simulink model "C2_sensor_backemf"  (Simulink 10.2)
settings: Solver=ode4  StartTime=0.0  StopTime=3  FixedStep=T_s  RelTol=1e-3
undefined symbols (not defined in the file): b_eq, beta_p, beta_v, g, i_rated, J_eq, k, L, L_l, m_l, N_adc, N_e, N_opt, R, R_sh, T_s, tau_m_rated, theta_0, V_adc
libraries: simulink x1
settings Model: Creator=ioannis  LastModifiedBy=mfocchi
settings DataIOCC: SaveFormat=Dataset  SignalLoggingSaveFormat=Dataset
settings OptimizationCC: LifeSpan=auto
settings DebuggingCC: UnderspecifiedInitializationDetection=Simplified  MergeDetectMultiDrivingBlocksExec=error  FcnCallInpInsideContextMsg=error  SFUnexpectedBacktrackingDiag=error  SFNoUnconditionalDefaultTransitionDiag=error  SFExecutionAtInitializationDiag=warning
settings HardwareCC: ProdBitPerPointer=64  ProdBitPerSizeT=64  ProdBitPerPtrDiffT=64  ProdLargestAtomicFloat=Float  ProdIntDivRoundTo=Zero  ProdEndianess=LittleEndian  ProdWordSize=64  ProdHWDeviceType=Intel->x86-64 (Windows64)
settings ModelReferenceCC: PropagateSignalLabelsOutOfModel=on
settings SFSimCC: SimUseLocalCustomCode=on
settings RTWCC: RTWUseLocalCustomCode=on
settings CodeAppCC: StateflowObjectComments=off
settings GRTTargetCC: TargetLangStandard=C99 (ISO)  CombineOutputUpdateFcns=on  GRTInterface=off
settings ConfigComp: CovMetricSettings=dwe  CovSaveCumulativeToWorkspaceVar=off  CovSaveSingleToWorkspaceVar=off  CovExternalEMLEnable=on

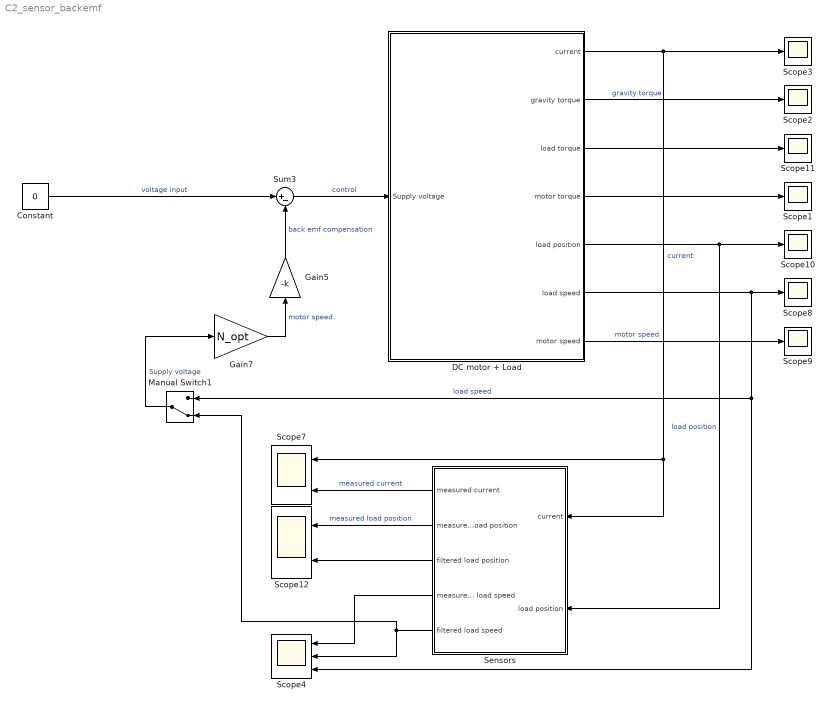
== system C2_sensor_backemf ==
  Constant : Constant  Value=0
  DC motor + Load : Subsystem
  Gain5 : Gain  Gain=-k
  Gain7 : Gain  Gain=N_opt
  Manual Switch1 : ManualSwitch  CurrentSetting=0
  Scope{1..3,8..11} (7 alike) : Scope
  Scope12 : Scope  NumInputPorts=2
  Scope4 : Scope  NumInputPorts=3
  Scope7 : Scope  NumInputPorts=2
  Sensors : Subsystem
  Sum3 : Sum  Inputs=|+-
  wires:
  DC motor + Load/6(load speed) -> Scope8/1, Scope4/3, Manual Switch1/1  "load speed"
  Sum3/1 -> DC motor + Load/1(Supply voltage)  "control"
  DC motor + Load/2(gravity torque) -> Scope2/1  "gravity torque"
  DC motor + Load/5(load position) -> Sensors/2(load position), Scope10/1  "load position"
  DC motor + Load/7(motor speed) -> Scope9/1  "motor speed"
  DC motor + Load/1(current) -> Sensors/1(current), Scope7/1, Scope3/1  "current"
  Constant/1 -> Sum3/1  "voltage input"
  DC motor + Load/3(load torque) -> Scope11/1
  DC motor + Load/4(motor torque) -> Scope1/1
  Sensors/2(measured load position) -> Scope12/1  "measured load position"
  Sensors/3(filtered load position) -> Scope12/2
  Sensors/4(measured load speed) -> Scope4/1
  Gain7/1 -> Gain5/1  "motor speed"
  Manual Switch1/1 -> Gain7/1  "Supply voltage"
  Sensors/5(filtered load speed) -> Scope4/2, Manual Switch1/2
  Sensors/1(measured current) -> Scope7/2  "measured current"
  Gain5/1 -> Sum3/2  "back emf compensation"

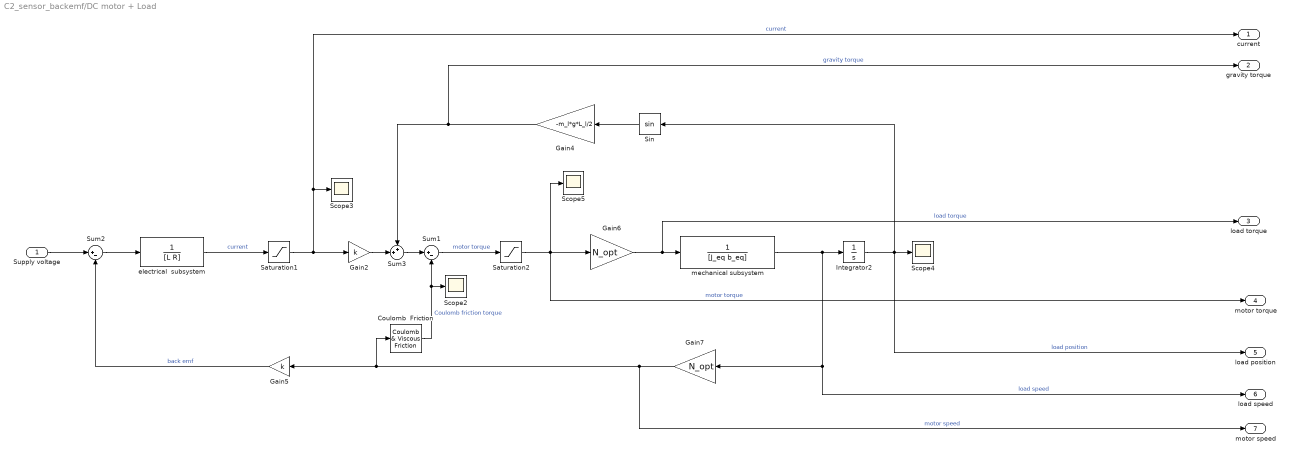
== system C2_sensor_backemf/DC motor + Load ==
  Supply voltage : Inport
  Coulomb  Friction : simulink/Discontinuities/Coulomb & Viscous Friction  offset=tau_c  gain=0
  Gain2 : Gain  Gain=k
  Gain4 : Gain  Gain=-m_l*g*L_l/2
  Gain5 : Gain  Gain=k
  Gain6 : Gain  Gain=N_opt
  Gain7 : Gain  Gain=N_opt
  Integrator2 : Integrator  InitialCondition=theta_0
  Saturation1 : Saturate  UpperLimit=i_rated  LowerLimit=-i_rated
  Saturation2 : Saturate  UpperLimit=tau_m_rated  LowerLimit=-tau_m_rated
  Scope{2..5} (4 alike) : Scope
  Sin : Trigonometry
  Sum1 : Sum  Inputs=|+-
  Sum2 : Sum  Inputs=|+-
  Sum3 : Sum  Inputs=++|
  electrical  subsystem : TransferFcn  Denominator=[L R]
  mechanical subsystem : TransferFcn  Denominator=[J_eq b_eq]
  current : Outport
  gravity torque : Outport  Port=2
  load torque : Outport  Port=3
  motor torque : Outport  Port=4
  load position : Outport  Port=5
  load speed : Outport  Port=6
  motor speed : Outport  Port=7
  wires:
  Sum2/1 -> electrical  subsystem/1
  Saturation2/1 -> motor torque/1, Scope5/1, Gain6/1  "motor torque"
  Sum3/1 -> Sum1/1
  Sum1/1 -> Saturation2/1  "motor torque"
  Sin/1 -> Gain4/1
  Gain5/1 -> Sum2/2  "back emf"
  electrical  subsystem/1 -> Saturation1/1  "current"
  Gain2/1 -> Sum3/2
  Gain6/1 -> load torque/1, mechanical subsystem/1  "load torque"
  mechanical subsystem/1 -> Gain7/1, load speed/1, Integrator2/1  "load speed"
  Supply voltage/1 -> Sum2/1
  Integrator2/1 -> Sin/1, load position/1, Scope4/1  "load position"
  Gain4/1 -> gravity torque/1, Sum3/1  "gravity torque"
  Saturation1/1 -> current/1, Scope3/1, Gain2/1  "current"
  Gain7/1 -> motor speed/1, Coulomb  Friction/1, Gain5/1  "motor speed"
  Coulomb  Friction/1 -> Sum1/2, Scope2/1  "Coulomb friction torque"

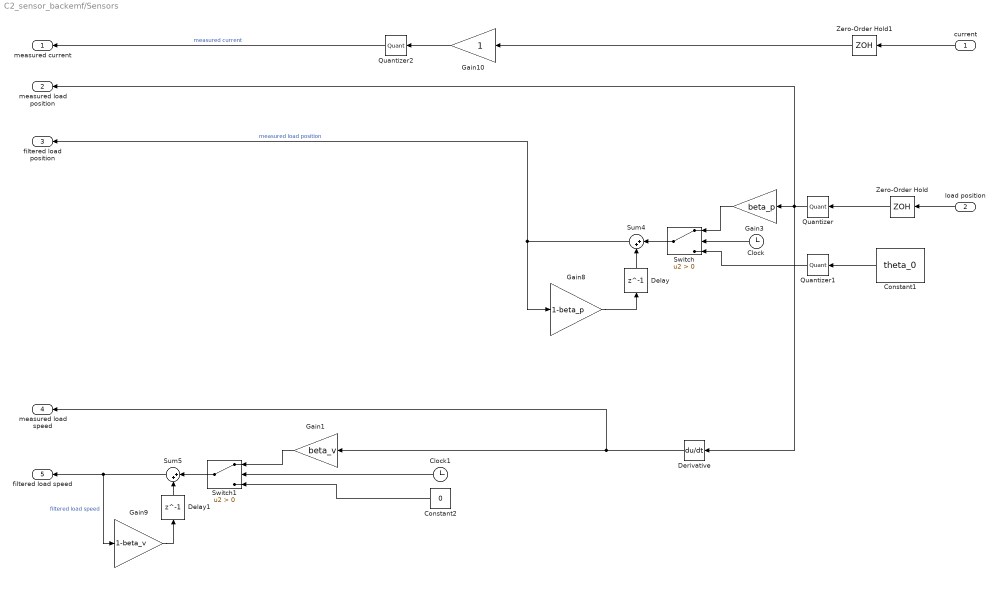
== system C2_sensor_backemf/Sensors ==
  current : Inport
  load position : Inport  Port=2
  Clock : Clock
  Clock1 : Clock
  Constant1 : Constant  Value=theta_0
  Constant2 : Constant  Value=0
  Delay : Delay  DelayLength=1  InitialCondition=0
  Delay1 : Delay  DelayLength=1  InitialCondition=0
  Derivative : Derivative
  Gain1 : Gain  Gain=beta_v
  Gain10 : Gain
  Gain3 : Gain  Gain=beta_p
  Gain8 : Gain  Gain=1-beta_p
  Gain9 : Gain  Gain=1-beta_v
  Quantizer : Quantizer  QuantizationInterval=2*pi/(2^N_e)
  Quantizer1 : Quantizer  QuantizationInterval=2*pi/(2^N_e)
  Quantizer2 : Quantizer  QuantizationInterval=V_adc/R_sh/(2^N_adc)
  Sum4 : Sum  Inputs=|++
  Sum5 : Sum  Inputs=|++
  Switch : Switch  Criteria=u2 > Threshold
  Switch1 : Switch  Criteria=u2 > Threshold
  Zero-Order Hold : ZeroOrderHold  SampleTime=T_s
  Zero-Order Hold1 : ZeroOrderHold  SampleTime=T_s
  measured current : Outport
  measured load position : Outport  Port=2
  filtered load position : Outport  Port=3
  measured load speed : Outport  Port=4
  filtered load speed : Outport  Port=5
  wires:
  Gain3/1 -> Switch/1
  Switch/1 -> Sum4/1
  Quantizer/1 -> Derivative/1, measured load position/1, Gain3/1
  Constant1/1 -> Quantizer1/1
  Delay/1 -> Sum4/2
  Quantizer1/1 -> Switch/3
  Quantizer2/1 -> measured current/1  "measured current"
  Gain10/1 -> Quantizer2/1
  Clock/1 -> Switch/2
  current/1 -> Zero-Order Hold1/1
  load position/1 -> Zero-Order Hold/1
  Sum4/1 -> filtered load position/1, Gain8/1  "measured load position"
  Gain8/1 -> Delay/1
  Zero-Order Hold/1 -> Quantizer/1
  Zero-Order Hold1/1 -> Gain10/1
  Clock1/1 -> Switch1/2
  Switch1/1 -> Sum5/1
  Sum5/1 -> filtered load speed/1, Gain9/1  "filtered load speed"
  Gain1/1 -> Switch1/1
  Delay1/1 -> Sum5/2
  Gain9/1 -> Delay1/1
  Constant2/1 -> Switch1/3
  Derivative/1 -> measured load speed/1, Gain1/1
